simulink model "Dyn_6DoF_v2_0_R2015B"  (R2015b)
settings: Solver=ode4  SolverMode=SingleTasking  StartTime=0.0  StopTime=simInit.TSIM  FixedStep=simInit.dt  MaxStep=simInit.dt  RelTol=1e-3
InitFcn:
  | close all
undefined symbols (not defined in the file): act, base_windspeed, constr, DE2019, DiscIntNeverNeededParam, ENVMT, Lbooth, loiterStates, omega_rate_max, params, simInit, T, winchParameter
libraries: simulink x41, simulink_extras x4, dspsigops x1
(part 5 of 6)

== matlab function Dyn_6DoF_v2_0_R2015B/AirborneSystem/6DoFDynamics/Subsystem/Estimations ==
  data: Ft input; F_a_B input; F_p_B input; v_k_B input; v_w_W input; mu_k output; Va output; mu_a output; alpha output; beta output; chi_a_dot_real output; gamma_a_dot_real output; M_OB input; longlat input; EULER input; pathangles_a output; pathangles_k output; v_k_O output; pos_W output; pos_O output; ENVMT parameter; DE2019 parameter; v_k_W output; h_tau input
% Copyright 2021 Delft University of Technology
%
% Licensed under the Apache License, Version 2.0 (the "License");
% you may not use this file except in compliance with the License.
% You may obtain a copy of the License at
%
%      http://www.apache.org/licenses/LICENSE-2.0
%
% Unless required by applicable law or agreed to in writing, software
% distributed under the License is distributed on an "AS IS" BASIS,
% WITHOUT WARRANTIES OR CONDITIONS OF ANY KIND, either express or implied.
% See the License for the specific language governing permissions and
% limitations under the License.

function [mu_k,Va, mu_a, alpha, beta, chi_a_dot_real,gamma_a_dot_real, ...
    pathangles_a, pathangles_k, v_k_O, pos_W, pos_O, v_k_W] = ...
    fcn(Ft, F_a_B, F_p_B, v_k_B, v_w_W,M_OB,longlat,EULER,...
    ENVMT, DE2019, h_tau)
%fcn - 6DoF dynamics estimations
%
% Inputs:
%    Ft      - Tether force magnitude at the kite
%    F_a_B   - Aerodynamic forces acting on kite in body reference frames
%    F_p_B   - Propulsion and brake forces acting on kite in body reference
%              frames 
%    v_k_B   - Kinetic velocity in body reference frame
%    M_OB    - Rotation matrix from body to inertial reference frame
%    longlat - Longtitude, latitude
%    EULER   - Euler angles
%    ENVMT   - Environment characteristics
%    DE2019  - Aircraft parameters
%    h_tau   - Height in tau reference frame
%
% Outputs:
%    mu_k              - Kinetic roll angle
%    Va                - Airspeed (magnitude)
%    mu_a              - Aerodynamic roll angle
%    alpha             - Pitch angle
%    beta              - Sideslip(yaw) angle
%    chi_a_dot_real    - rate of change in aerodynamic course heading
%    gamma_a_dot_real  - rate of change in aerodynamic path angle
%    pathangles_a      - Aerodynamic course heading and path angle
%    pathangles_k      - Kinetic course heading and path angle
%    v_k_O             - Kinetic velocity in inertial reference frame
%    pos_W             - Kite position in wind reference frame
%    pos_O             - Kite position in inertial reference frame
%    v_k_W             - Kinetic velocity in wind reference frame
%
% Author: Sebastian Rapp, Ph.D., Revised by: Dylan Eijkelhof, M.Sc.
% Delft University of Technology
% email address: d.eijkelhof@tudelft.nl
% December 2019; Last revision: 19-March-2021

%-------------	BEGIN CODE	--------------
% Preallocate variables
mu_k             = 0;
Va               = 0;
mu_a             = 0;
alpha            = 0; 
beta             = 0;
chi_a_dot_real   = 0;
gamma_a_dot_real = 0;
pathangles_a     = zeros(2,1);
pathangles_k     = zeros(2,1); 
M_B2ABar         = zeros(3,3);

long = longlat(1);
lat  = longlat(2);

M_WO = [cos(ENVMT.windDirection_rad), sin(ENVMT.windDirection_rad), 0;
        sin(ENVMT.windDirection_rad), -cos(ENVMT.windDirection_rad), 0;
        0, 0, -1];
    
pos_W = [cos(long)*cos(lat);
         sin(long)*cos(lat);
         sin(lat)]*abs(h_tau);
    
pos_O = M_WO'*pos_W;   
v_k_O = M_OB*v_k_B;
v_k_W =  M_WO*v_k_O;

v_a_W = v_k_W - v_w_W;
Va = norm(v_a_W);

v_a_O = transformFromWtoO(ENVMT.windDirection_rad, v_a_W);
v_a_B = M_OB' * v_a_O;

chi_k        = atan2( v_k_O(2), v_k_O(1) );
gamma_k      = -asin( v_k_O(3)/norm(v_k_O) );
pathangles_k = [chi_k; gamma_k];

chi_a        = atan2( v_a_O(2), v_a_O(1) );
gamma_a      = -asin( v_a_O(3)/norm(v_a_O) );
pathangles_a = [chi_a; gamma_a];

% Estimation of aerodynamic angles 
alpha = atan2( v_a_B(3), v_a_B(1) );
beta  = asin( v_a_B(2)/norm(v_a_B) );
mu_a  = asin( max( min( (cos(EULER(2))*sin(EULER(1)))/(cos(gamma_a)*cos(beta)) ...
    + tan(gamma_a) * tan(beta), 1),-1) ); 

beta_k = atan2( v_k_B(2), norm(v_k_B) );
mu_k   = asin( max( min( (cos(EULER(2))*sin(EULER(1)))/(cos(gamma_k)*cos(beta_k)) ...
    + tan(gamma_k) * tan(beta_k), 1),-1) ); 

c_m = cos(mu_a);
s_m = sin(mu_a);

c_a = cos(alpha);
s_a = sin(alpha);

c_b = cos(beta);
s_b = sin(beta);

M_B2ABar(1,1) = c_a*c_b;
M_B2ABar(1,2) = s_b;
M_B2ABar(1,3) = s_a*c_b;
M_B2ABar(2,1) = -c_a*s_b*c_m+s_a*s_m;
M_B2ABar(2,2) = c_b*c_m;
M_B2ABar(2,3) = -s_a*s_b*c_m-s_m*c_a;
M_B2ABar(3,1) = -c_a*s_b*s_m-s_a*c_m;
M_B2ABar(3,2) = c_b*s_m;
M_B2ABar(3,3) = -s_a*s_b*s_m+c_a*c_m;

% Estimtion of chi_a_dot and gamma_a_dot
c_chia = cos(chi_a);
s_chia = sin(chi_a);

c_gama = cos(gamma_a);
s_gama = sin(gamma_a);

M_ABar2O = zeros(3,3);

M_ABar2O(1,1) = c_chia*c_gama;
M_ABar2O(2,1) = s_chia*c_gama;
M_ABar2O(3,1) = -s_gama;
M_ABar2O(1,2) = -s_chia;
M_ABar2O(2,2) = c_chia;
M_ABar2O(3,2) = 0;
M_ABar2O(1,3) = c_chia*s_gama;
M_ABar2O(2,3) = s_chia*s_gama;
M_ABar2O(3,3) = c_gama;


F_g_t_Abar  = M_ABar2O' * ( [0;0;DE2019.mass*ENVMT.g] -Ft*pos_O/norm(pos_O) );
F_ap_B      = M_B2ABar * (F_a_B+F_p_B);
f_y         = F_ap_B(2) + F_g_t_Abar(2); 
f_z         = F_ap_B(3) + F_g_t_Abar(3);

chi_a_dot_real   = 1/cos(gamma_a)/Va/DE2019.mass  * (f_y);
gamma_a_dot_real = -1/Va/DE2019.mass * (f_z);

%-------------	END CODE	--------------
end

== matlab function Dyn_6DoF_v2_0_R2015B/AirborneSystem/6DoFDynamics/Subsystem/MATLAB Function2 ==
  data: v_k_B input; DE2019 parameter; F_a_B input; F_p_B input; ENVMT parameter; F_t_W input; Torques_B input; vel_k_W input; omega_OB_B input; longlat input; EULER input; h_tau input; vel_K_B_dot output; M_OB output; omega_OB_B_dot output; longlat_dot output; eta_EULER_dot output; h_tau_dot output
% Copyright 2021 Delft University of Technology
%
% Licensed under the Apache License, Version 2.0 (the "License");
% you may not use this file except in compliance with the License.
% You may obtain a copy of the License at
%
%      http://www.apache.org/licenses/LICENSE-2.0
%
% Unless required by applicable law or agreed to in writing, software
% distributed under the License is distributed on an "AS IS" BASIS,
% WITHOUT WARRANTIES OR CONDITIONS OF ANY KIND, either express or implied.
% See the License for the specific language governing permissions and
% limitations under the License.

function [vel_K_B_dot, M_OB, omega_OB_B_dot, longlat_dot, ...
    eta_EULER_dot, h_tau_dot] = fcn(v_k_B, DE2019, F_a_B, F_p_B ,...
    ENVMT, F_t_W, Torques_B, vel_k_W, omega_OB_B, longlat, EULER, h_tau)
%fcn - 6DoF dynamics
%
% Inputs:
%    v_k_B      - Kinetic velocity in body reference frame
%    DE2019     - Aircraft parameters
%    F_a_B      - Aerodynamic forces acting on kite in body reference frame
%    F_p_B      - Propulsion and brake forces acting on kite in body
%                 reference frame
%    ENVMT      - Environment characteristics
%    F_t_W      - Tether force pulling at the kite
%    Torques_B  - Roll, pitch and yaw moments in body reference frame
%    vel_k_W    - Kinetic velocity in wind reference frame
%    omega_OB_B - Roll, pitch and yaw rates
%    longlat    - Longtitude, latitude
%    EULER      - Euler angles
%    h_tau      - Height in tau reference frame
%
% Outputs:
%    vel_K_B_dot    - Rate of change in kinetic velocity in body reference
%                     frame
%    M_OB           - Rotation matrix from body to inertial reference frame
%    omega_OB_B_dot - Roll, pitch and yaw accellerations
%    longlat_dot    - Rate of change of longtitude, latitude
%    eta_EULER_dot	- Rate of change of euler angles
%    h_tau_dot      - Rate of change of height in tau reference frame
%
%
% Author: Sebastian Rapp, Ph.D., Revised by: Dylan Eijkelhof, M.Sc.
% Delft University of Technology
% email address: d.eijkelhof@tudelft.nl
% December 2019; Last revision: 19-March-2021

%-------------	BEGIN CODE	--------------
% Preallocate variables
omega_OB_B_dot = zeros(3,1);
eta_EULER_dot  = zeros(3,1);
longlat_dot    = zeros(2,1);
vel_K_B_dot    = zeros(3,1);

c_psi = cos(EULER(3));
s_psi = sin(EULER(3));

c_theta = cos(EULER(2));
s_theta = sin(EULER(2));

c_phi = cos(EULER(1));
s_phi = sin(EULER(1)); 

M_OB = [ c_psi*c_theta, c_psi*s_theta*s_phi-s_psi*c_phi, c_psi*s_theta*c_phi+s_psi*s_phi;
         s_psi*c_theta, s_psi*s_theta*s_phi+c_psi*c_phi, s_psi*s_theta*c_phi-c_psi*s_phi;
        -s_theta, c_theta*s_phi, c_theta*c_phi];

long = longlat(1);
lat  = longlat(2);

F_g_O = [0;0;DE2019.mass*ENVMT.g];
F_t_O = transformFromOtoW( ENVMT.windDirection_rad, F_t_W);

%Forces to body fixed frame
F_g_t_B  = M_OB'*(F_g_O+F_t_O); 
Forces_B = F_a_B + F_g_t_B + F_p_B ;

p=omega_OB_B(1);
q=omega_OB_B(2);
r=omega_OB_B(3);

u=v_k_B(1);
v=v_k_B(2);
w=v_k_B(3);
vel_K_B_dot = [r*v-q*w + 1/DE2019.mass * Forces_B(1);
               p*w-r*u + 1/DE2019.mass * Forces_B(2);
               q*u-p*v + 1/DE2019.mass * Forces_B(3)];

c_theta = cos(EULER(2));
s_theta = sin(EULER(2));

c_phi = cos(EULER(1));
s_phi = sin(EULER(1)); 

eta_EULER_dot = [1 s_phi*s_theta/c_theta c_phi*s_theta/c_theta;
                 0 c_phi -s_phi; 
                 0 s_phi/c_theta c_phi/c_theta]*omega_OB_B;

Gamma  = DE2019.Jx*DE2019.Jz-DE2019.Jxz^2;
Gamma1 = (DE2019.Jxz*(DE2019.Jx - DE2019.Jy + DE2019.Jz ))/Gamma;
Gamma2 = (DE2019.Jz * (DE2019.Jz - DE2019.Jy) + DE2019.Jxz^2)/Gamma;
Gamma3 = DE2019.Jz/Gamma;
Gamma4 = DE2019.Jxz/Gamma;
Gamma5 = (DE2019.Jz - DE2019.Jx)/DE2019.Jy;
Gamma6 = DE2019.Jxz / DE2019.Jy;
Gamma7 = ((DE2019.Jx - DE2019.Jy)*DE2019.Jx + DE2019.Jxz^2 )/Gamma;
Gamma8 = DE2019.Jx / Gamma;

omega_OB_B_dot = [Gamma1 * p * q - Gamma2 * q * r + Gamma3 * Torques_B(1) + Gamma4 * Torques_B(3);
    Gamma5 * p * r - Gamma6 * (p^2 - r^2) + 1/DE2019.Jy *Torques_B(2);
     Gamma7 * p * q - Gamma1 * q * r + Gamma4 * Torques_B(1) + Gamma8 * Torques_B(3)];

%% Position propagation
sin_lat  = sin(lat);
sin_long = sin(long);
cos_lat  = cos(lat);
cos_long = cos(long);
 
M_tauW = [-sin_lat*cos_long, -sin_lat*sin_long,cos_lat;
    -sin_long, cos_long, 0;
    -cos_lat*cos_long, -cos_lat*sin_long, -sin_lat];

v_k_tau = M_tauW*vel_k_W;

long_dot = v_k_tau(2)/( abs(h_tau)*cos(lat));
lat_dot  = v_k_tau(1)/abs(h_tau);

h_tau_dot = -v_k_tau(3);

longlat_dot = [long_dot;
               lat_dot];

%-------------	END CODE	--------------
end

== matlab function Dyn_6DoF_v2_0_R2015B/AirborneSystem/FlightControlSystem/AttitudeAndRateLoop/AttitudeController/InversionAttitude ==
  data: omega_OB_B_cmd output size=[3,1]; mu_a input size=1; alpha input size=1; beta input size=1; nu_mu_a input size=1; nu_alpha_a input size=1; nu_beta_a input size=1; chi_a_dot_real input size=1; gamma_a_dot_real input size=1; gamma_a input; nu_hat output; constr parameter
% Copyright 2021 Delft University of Technology
%
% Licensed under the Apache License, Version 2.0 (the "License");
% you may not use this file except in compliance with the License.
% You may obtain a copy of the License at
%
%      http://www.apache.org/licenses/LICENSE-2.0
%
% Unless required by applicable law or agreed to in writing, software
% distributed under the License is distributed on an "AS IS" BASIS,
% WITHOUT WARRANTIES OR CONDITIONS OF ANY KIND, either express or implied.
% See the License for the specific language governing permissions and
% limitations under the License.

function [omega_OB_B_cmd, nu_hat]  = Attitude_inv( mu_a, alpha, beta, nu_mu_a,...
                                    nu_alpha_a, nu_beta_a, chi_a_dot_real,...
                                    gamma_a_dot_real, gamma_a, constr)
%Attitude_inv - Inverse attitude from error to actual
%
% Inputs:
%    mu_a               - Actual roll angle
%    alpha              - Actual pitch angle
%    beta               - Actual yaw angle
%    nu_mu_a            - Roll angle error w.r.t. actual with controller gains
%    nu_alpha_a         - Pitch angle error w.r.t. actual with controller gains
%    nu_beta_a          - Yaw angle error w.r.t. actual with controller gains
%    chi_a_dot_real     - Rate of change of course heading
%    gamma_a_dot_real   - Rate of change of path angle
%    gamma_a            - Actual aerodynamic path angle
%    constr             - Aircraft manoeuvre constraints
%
% Outputs:
%    omega_OB_B_cmd     - Commanded roll, pitch and yaw rates
%    nu_hat             - Expected error
%
%
% Author: Sebastian Rapp, Ph.D., Revised by: Dylan Eijkelhof, M.Sc.
% Delft University of Technology
% email address: d.eijkelhof@tudelft.nl
% December 2019; Last revision: 19-March-2021

%-------------	BEGIN CODE	--------------

c_m = cos(mu_a);
s_m = sin(mu_a);

c_a = cos(alpha);
s_a = sin(alpha);

c_b = cos(beta);
s_b = sin(beta);

M_B2ABar = zeros(3,3);

M_B2ABar(1,1) = c_a*c_b;
M_B2ABar(1,2) = s_b;
M_B2ABar(1,3) = s_a*c_b;
M_B2ABar(2,1) = -c_a*s_b*c_m+s_a*s_m;
M_B2ABar(2,2) = c_b*c_m;
M_B2ABar(2,3) = -s_a*s_b*c_m-s_m*c_a;
M_B2ABar(3,1) = -c_a*s_b*s_m-s_a*c_m;
M_B2ABar(3,2) = c_b*s_m;
M_B2ABar(3,3) = -s_a*s_b*s_m+c_a*c_m;


%% Inversion 

omega_OAbar_Abar = [-chi_a_dot_real*sin(gamma_a); 
                     gamma_a_dot_real; 
                     chi_a_dot_real*cos(gamma_a)];
                 
omega_OAbar_B = M_B2ABar'*omega_OAbar_Abar;
omega_OB_B_cmd =  [cos(alpha)*cos(beta) * nu_mu_a + nu_beta_a*sin(alpha); 
                  sin(beta)*nu_mu_a+nu_alpha_a;
                    sin(alpha)*cos(beta)*nu_mu_a - cos(alpha)*nu_beta_a] + omega_OAbar_B;

omega_OB_B_cmd_sat = max( min( omega_OB_B_cmd , constr.max_rates_B), -constr.max_rates_B ); 

% Expected pseudo-control
omega_AB_B = omega_OB_B_cmd_sat - M_B2ABar'*( [-chi_a_dot_real*sin(gamma_a);
                         gamma_a_dot_real; 
                         chi_a_dot_real*cos(gamma_a)]);
nu_x_hat = ( c_a*omega_AB_B(1) + s_a * omega_AB_B(3)  )/cos( beta );
nu_y_hat = -s_b*nu_x_hat  + omega_AB_B(2); 
nu_z_hat = ( omega_AB_B(1)*s_a - omega_AB_B(3) * c_a );
nu_hat = [nu_x_hat; nu_y_hat; nu_z_hat];

end

== matlab function Dyn_6DoF_v2_0_R2015B/AirborneSystem/FlightControlSystem/AttitudeAndRateLoop/RateLoop/ControlAllocation/allocation ==
  data: dC_pqr input; Delta_deltas output; alpha input; DE2019 parameter
% Copyright 2021 Delft University of Technology
%
% Licensed under the Apache License, Version 2.0 (the "License");
% you may not use this file except in compliance with the License.
% You may obtain a copy of the License at
%
%      http://www.apache.org/licenses/LICENSE-2.0
%
% Unless required by applicable law or agreed to in writing, software
% distributed under the License is distributed on an "AS IS" BASIS,
% WITHOUT WARRANTIES OR CONDITIONS OF ANY KIND, either express or implied.
% See the License for the specific language governing permissions and
% limitations under the License.

function Delta_deltas = fcn(dC_pqr, alpha, DE2019)
%Attitude_inv - Allocation matrix from moment increments to surface increments.
%
% Inputs:
%    dC_pqr        - Delta roll, pitch and yaw coefficients
%    alpha         - Actual pitch angle
%    DE2019        - Aircraft parameters
%
% Outputs:
%    Delta_deltas  - Delta actuator deflections
%
% Author: Sebastian Rapp, Ph.D., Revised by: Dylan Eijkelhof, M.Sc.
% Delft University of Technology
% email address: d.eijkelhof@tudelft.nl
% December 2019; Last revision: 19-March-2021

%-------------	BEGIN CODE	--------------
 
Cl_deltaA =DE2019.Cl_deltaA_0 + DE2019.Cl_deltaA_alpha * alpha + DE2019.Cl_deltaA_alpha2 * alpha^2;
Cl_deltaR =DE2019.Cl_deltaR_0 + DE2019.Cl_deltaR_alpha * alpha + DE2019.Cl_deltaR_alpha2 * alpha^2;                                 
 
Cm_deltaA =DE2019.Cm_deltaA_0 + DE2019.Cm_deltaA_alpha * alpha + DE2019.Cm_deltaA_alpha2 * alpha^2;  
Cm_deltaE = DE2019.Cm_deltaE_0  + DE2019.Cm_deltaE_alpha * alpha + DE2019.Cm_deltaE_alpha2 * alpha^2; 
 
Cn_deltaA =DE2019.Cn_deltaA_0 + DE2019.Cn_deltaA_alpha * alpha + DE2019.Cn_deltaA_alpha2 * alpha^2;  
Cn_deltaR =DE2019.Cn_deltaR_0 + DE2019.Cn_deltaR_alpha * alpha + DE2019.Cn_deltaR_alpha2 * alpha^2;
 
Ba = [[Cl_deltaA,0,Cl_deltaR];[Cm_deltaA,Cm_deltaE,0];[Cn_deltaA,0,Cn_deltaR]];
 
Delta_deltas = Ba\dC_pqr;

%-------------	END CODE	--------------
 
end

== matlab function Dyn_6DoF_v2_0_R2015B/AirborneSystem/ForcesAndTorques/aerodynamic forces FSI/Wing Aero/If Action Subsystem/MATLAB Function ==
  data: u input; y output
% Copyright 2021 Delft University of Technology
%
% Licensed under the Apache License, Version 2.0 (the "License");
% you may not use this file except in compliance with the License.
% You may obtain a copy of the License at
%
%      http://www.apache.org/licenses/LICENSE-2.0
%
% Unless required by applicable law or agreed to in writing, software
% distributed under the License is distributed on an "AS IS" BASIS,
% WITHOUT WARRANTIES OR CONDITIONS OF ANY KIND, either express or implied.
% See the License for the specific language governing permissions and
% limitations under the License.

function y = placeholder(u)

y = zeros(6,1);

== matlab function Dyn_6DoF_v2_0_R2015B/RequirementModelsAndLogging/MATLAB Function ==
  data: time input; eul input; stop_flag output; eul_old input
% Copyright 2021 Delft University of Technology
%
% Licensed under the Apache License, Version 2.0 (the "License");
% you may not use this file except in compliance with the License.
% You may obtain a copy of the License at
%
%      http://www.apache.org/licenses/LICENSE-2.0
%
% Unless required by applicable law or agreed to in writing, software
% distributed under the License is distributed on an "AS IS" BASIS,
% WITHOUT WARRANTIES OR CONDITIONS OF ANY KIND, either express or implied.
% See the License for the specific language governing permissions and
% limitations under the License.

function stop_flag = fcn(time, eul,eul_old)
phi = eul(1);
theta = eul(2);
% psi = eul(3);

phi_old = eul_old(1);
theta_old = eul_old(2);
% psi_old = eul_old(3);

if time>40
    if ((phi>pi/2 || phi<-pi/2) && sign(phi) ~= sign(phi_old))
        stop_flag = 1;
    elseif ((theta>pi/2 || theta<-pi/2) && sign(theta) ~= sign(theta_old))
        stop_flag = 1; 
%     elseif ((psi>pi/2 || psi<-pi/2) && sign(psi) ~= sign(psi_old))
%         stop_flag = 1; 
    else
        stop_flag = 0;
    end
else
    stop_flag = 0;
end
end

== matlab function Dyn_6DoF_v2_0_R2015B/RequirementModelsAndLogging/MATLAB Function1 ==
  data: Lift output; F_a_B input; Drag output; AoA input
% Copyright 2021 Delft University of Technology
%
% Licensed under the Apache License, Version 2.0 (the "License");
% you may not use this file except in compliance with the License.
% You may obtain a copy of the License at
%
%      http://www.apache.org/licenses/LICENSE-2.0
%
% Unless required by applicable law or agreed to in writing, software
% distributed under the License is distributed on an "AS IS" BASIS,
% WITHOUT WARRANTIES OR CONDITIONS OF ANY KIND, either express or implied.
% See the License for the specific language governing permissions and
% limitations under the License.

function [Lift, Drag]  = estimate_drag(F_a_B, AoA)
%estimate_drag - Transform drag from B to A reference frame
%
% Inputs:
%    F_a_B     - Aerodynamic forces in body reference frame
%    AoA       - Angle of Attack
%
% Outputs:
%    Drag    - Drag force
%
% Example: 
%    [Drag] = estimate_drag(F_a_B, AoA)
%
% Author: Sebastian Rapp, Ph.D., Revised by: Dylan Eijkelhof, M.Sc.
% Delft University of Technology
% email address: s.rapp@tudelft.nl
% email address: d.eijkelhof@tudelft.nl
% December 2019; Last revision: 06-October-2020

%-------------	BEGIN CODE	--------------

F_a_A = [cos(AoA), 0, sin(AoA);
    0, 1, 0; 
    -sin(AoA), 0, cos(AoA)] * F_a_B;

Lift = -F_a_A(3);
Drag = -F_a_A(1);

%-------------	 END CODE	--------------

end

== matlab function Dyn_6DoF_v2_0_R2015B/AirborneSystem/FlightControlSystem/PathFollowingController_SS_3/FlightOnFlatEarth (Retraction&Loitering)/CalculateAttitudeCmds/FlightPathLoopRetraction_Aerodynamic/FlightpathReferenceModels/SecondOrderReferenceModel_course/wrapto2pi ==
  data: u input; y output
% Copyright 2021 Delft University of Technology
%
% Licensed under the Apache License, Version 2.0 (the "License");
% you may not use this file except in compliance with the License.
% You may obtain a copy of the License at
%
%      http://www.apache.org/licenses/LICENSE-2.0
%
% Unless required by applicable law or agreed to in writing, software
% distributed under the License is distributed on an "AS IS" BASIS,
% WITHOUT WARRANTIES OR CONDITIONS OF ANY KIND, either express or implied.
% See the License for the specific language governing permissions and
% limitations under the License.

function y = wrap_to_2pi(u)
u = mod(u, 2*pi); 
if u > pi 
    du = mod(u,pi);
    y = -pi+du; 
elseif u < -pi 
    du = mod(u,-pi); 
    y = pi+du;
else
    y = u; 
end
end

== matlab function Dyn_6DoF_v2_0_R2015B/Environment_SS_5/MATLAB Function1 ==
  data: v_w_u input; v_w_p_mat output
% Copyright 2021 Delft University of Technology
%
% Licensed under the Apache License, Version 2.0 (the "License");
% you may not use this file except in compliance with the License.
% You may obtain a copy of the License at
%
%      http://www.apache.org/licenses/LICENSE-2.0
%
% Unless required by applicable law or agreed to in writing, software
% distributed under the License is distributed on an "AS IS" BASIS,
% WITHOUT WARRANTIES OR CONDITIONS OF ANY KIND, either express or implied.
% See the License for the specific language governing permissions and
% limitations under the License.

function v_w_p_mat = fcn(v_w_u)

v_w_p_mat = zeros( 3, length( v_w_u) );
v_w_p_mat(1,:) = v_w_u';

== matlab function Dyn_6DoF_v2_0_R2015B/AirborneSystem/FlightControlSystem/AirspeedController_SS_1/Airspeed_Brake/FeedforwardPart ==
  data: gamma input; BF output; nu_V input; ENVMT parameter; Drag_force input; DE2019 parameter
% Copyright 2021 Delft University of Technology
%
% Licensed under the Apache License, Version 2.0 (the "License");
% you may not use this file except in compliance with the License.
% You may obtain a copy of the License at
%
%      http://www.apache.org/licenses/LICENSE-2.0
%
% Unless required by applicable law or agreed to in writing, software
% distributed under the License is distributed on an "AS IS" BASIS,
% WITHOUT WARRANTIES OR CONDITIONS OF ANY KIND, either express or implied.
% See the License for the specific language governing permissions and
% limitations under the License.

function BF = feedforward_brake(gamma, nu_V,  ENVMT, Drag_force, DE2019)
%feedforward_brake - Brake force calculation for velocity decrease
%
% Inputs:
%    gamma      - Path angle (glideslope)
%    nu_V       - Controlled velocity parameter
%    ENVMT      - Environmental characteristics
%    Drag_force	- Drag
%    DE2019     - Aircraft characteristics
%
% Outputs:
%    BF          - Brake force
%
% Example: 
%    BF = feedforward_thrust(gamma, nu_V,  ENVMT, Drag_force, DE2019)
%
% Author: Sebastian Rapp, Ph.D., Revised by: Dylan Eijkelhof, M.Sc.
% Delft University of Technology
% email address: s.rapp@tudelft.nl
% email address: d.eijkelhof@tudelft.nl
% December 2019; Last revision: 06-October-2020

%-------------	BEGIN CODE	--------------

BF = DE2019.mass * ( ENVMT.g * sin(gamma) + nu_V ) + Drag_force; % required thrust

%-------------	 END CODE	--------------
end

== stateflow chart Dyn_6DoF_v2_0_R2015B/GroundSystem_SS_6/GroundControl/Select_init_sol_for_pathfollowing ==
  state Init
    entry: sol_init = x;
  state Pumping
    entry: sol_init = transition_phi;
  (default) -> Init
  Init -> Pumping : [fm == 6]
  data: x input; fm input; sol_init output; transition_phi input

== matlab function Dyn_6DoF_v2_0_R2015B/AirborneSystem/FlightControlSystem/AirspeedController_SS_1/Airspeed_Brake/MATLAB Function ==
  data: F_a_B input; Drag output; AoA input
% Copyright 2021 Delft University of Technology
%
% Licensed under the Apache License, Version 2.0 (the "License");
% you may not use this file except in compliance with the License.
% You may obtain a copy of the License at
%
%      http://www.apache.org/licenses/LICENSE-2.0
%
% Unless required by applicable law or agreed to in writing, software
% distributed under the License is distributed on an "AS IS" BASIS,
% WITHOUT WARRANTIES OR CONDITIONS OF ANY KIND, either express or implied.
% See the License for the specific language governing permissions and
% limitations under the License.

function Drag  = estimate_drag(F_a_B, AoA)
%estimate_drag - Transform drag from B to A reference frame
%
% Inputs:
%    F_a_B     - Aerodynamic forces in body reference frame
%    AoA       - Angle of Attack
%
% Outputs:
%    Drag    - Drag force
%
% Example: 
%    [Drag] = estimate_drag(F_a_B, AoA)
%
% Author: Sebastian Rapp, Ph.D., Revised by: Dylan Eijkelhof, M.Sc.
% Delft University of Technology
% email address: s.rapp@tudelft.nl
% email address: d.eijkelhof@tudelft.nl
% December 2019; Last revision: 06-October-2020

%-------------	BEGIN CODE	--------------

F_a_A = [cos(AoA), 0, sin(AoA);
    0, 1, 0; 
    -sin(AoA), 0, cos(AoA)] * F_a_B;

Drag = -F_a_A(1);

%-------------	 END CODE	--------------

end

== matlab function Dyn_6DoF_v2_0_R2015B/AirborneSystem/FlightControlSystem/AirspeedController_SS_1/Airspeed_Brake/hedging ==
  data: Drag_force input; gamma input; nu_V output; BF input; ENVMT parameter; DE2019 parameter
% Copyright 2021 Delft University of Technology
%
% Licensed under the Apache License, Version 2.0 (the "License");
% you may not use this file except in compliance with the License.
% You may obtain a copy of the License at
%
%      http://www.apache.org/licenses/LICENSE-2.0
%
% Unless required by applicable law or agreed to in writing, software
% distributed under the License is distributed on an "AS IS" BASIS,
% WITHOUT WARRANTIES OR CONDITIONS OF ANY KIND, either express or implied.
% See the License for the specific language governing permissions and
% limitations under the License.

function nu_V = hedgingV(Drag_force, gamma, BF, ENVMT, DE2019)

%hedgingV
%
% Inputs:
%    Drag_force	- Drag
%    gamma      - Path angle (glideslope)
%    BF         - Brake force
%    ENVMT      - Environmental characteristics
%    DE2019     - Aircraft characteristics
%
% Outputs:
%    nu_V       - Controlled velocity parameter
%
% Example: 
%    nu_V = hedgingV(Drag_force, gamma, BF, ENVMT, DE2019)
%
% Author: Sebastian Rapp, Ph.D., Revised by: Dylan Eijkelhof, M.Sc.
% Delft University of Technology
% email address: s.rapp@tudelft.nl
% email address: d.eijkelhof@tudelft.nl
% December 2019; Last revision: 06-October-2020

%-------------	BEGIN CODE	--------------

nu_V = (BF-Drag_force)/DE2019.mass - ENVMT.g * sin(gamma); 

%-------------	 END CODE	--------------
end

== matlab function Dyn_6DoF_v2_0_R2015B/AirborneSystem/FlightControlSystem/AirspeedController_SS_1/Airspeed_Control/FeedforwardPart ==
  data: gamma input; T output; nu_V input; ENVMT parameter; Drag_force input; DE2019 parameter
% Copyright 2021 Delft University of Technology
%
% Licensed under the Apache License, Version 2.0 (the "License");
% you may not use this file except in compliance with the License.
% You may obtain a copy of the License at
%
%      http://www.apache.org/licenses/LICENSE-2.0
%
% Unless required by applicable law or agreed to in writing, software
% distributed under the License is distributed on an "AS IS" BASIS,
% WITHOUT WARRANTIES OR CONDITIONS OF ANY KIND, either express or implied.
% See the License for the specific language governing permissions and
% limitations under the License.

function T = feedforward_thrust(gamma, nu_V,  ENVMT, Drag_force, DE2019)
%feedforward_thrust - Thrust calculation for velocity initialisation
%
% Inputs:
%    gamma      - Path angle (glideslope)
%    nu_V       - Controlled velocity parameter
%    ENVMT      - Environmental characteristics
%    Drag_force	- Drag
%    DE2019     - Aircraft characteristics
%
% Outputs:
%    T          - Thrust force
%
% Example: 
%    T = feedforward_thrust(gamma, nu_V,  ENVMT, Drag_force, DE2019)
%
% Author: Sebastian Rapp, Ph.D., Revised by: Dylan Eijkelhof, M.Sc.
% Delft University of Technology
% email address: s.rapp@tudelft.nl
% email address: d.eijkelhof@tudelft.nl
% December 2019; Last revision: 06-October-2020

%-------------	BEGIN CODE	--------------

T = DE2019.mass * ( ENVMT.g * sin(gamma) + nu_V ) + Drag_force; % required thrust

% Based on the quotient of commmanded to max. available thrust
% F_T_max = ENVMT.rhos * DE2019.S_prop * DE2019.C_prop * DE2019.k_motor * (DE2019.k_motor - Va);
% delta_t = T/F_T_max; 

%-------------	 END CODE	--------------
end

== matlab function Dyn_6DoF_v2_0_R2015B/AirborneSystem/FlightControlSystem/AirspeedController_SS_1/Airspeed_Control/MATLAB Function ==
  data: F_a_B input; Drag output; AoA input
% Copyright 2021 Delft University of Technology
%
% Licensed under the Apache License, Version 2.0 (the "License");
% you may not use this file except in compliance with the License.
% You may obtain a copy of the License at
%
%      http://www.apache.org/licenses/LICENSE-2.0
%
% Unless required by applicable law or agreed to in writing, software
% distributed under the License is distributed on an "AS IS" BASIS,
% WITHOUT WARRANTIES OR CONDITIONS OF ANY KIND, either express or implied.
% See the License for the specific language governing permissions and
% limitations under the License.

function Drag = estimate_drag(F_a_B, AoA)

%estimate_drag - Transform drag from B to A reference frame
%
% Inputs:
%    F_a_B     - Aerodynamic forces in body reference frame
%    AoA       - Angle of Attack
%
% Outputs:
%    Drag    - Drag force
%
% Example: 
%    Drag = estimate_drag(F_a_B, AoA)
%
% Author: Sebastian Rapp, Ph.D., Revised by: Dylan Eijkelhof, M.Sc.
% Delft University of Technology
% email address: s.rapp@tudelft.nl
% email address: d.eijkelhof@tudelft.nl
% December 2019; Last revision: 06-October-2020

%-------------	BEGIN CODE	--------------

F_a_A = [cos(AoA), 0, sin(AoA);
    0, 1, 0; 
    -sin(AoA), 0, cos(AoA)] * F_a_B;

Drag = -F_a_A(1);

%-------------	 END CODE	--------------
end

== matlab function Dyn_6DoF_v2_0_R2015B/AirborneSystem/FlightControlSystem/AirspeedController_SS_1/Airspeed_Control/hedging ==
  data: Drag_force input; gamma input; nu_V output; T input; ENVMT parameter; DE2019 parameter
% Copyright 2021 Delft University of Technology
%
% Licensed under the Apache License, Version 2.0 (the "License");
% you may not use this file except in compliance with the License.
% You may obtain a copy of the License at
%
%      http://www.apache.org/licenses/LICENSE-2.0
%
% Unless required by applicable law or agreed to in writing, software
% distributed under the License is distributed on an "AS IS" BASIS,
% WITHOUT WARRANTIES OR CONDITIONS OF ANY KIND, either express or implied.
% See the License for the specific language governing permissions and
% limitations under the License.

function nu_V = hedgingV(Drag_force, gamma, T, ENVMT, DE2019)

%hedgingV
%
% Inputs:
%    Drag_force	- Drag
%    gamma      - Path angle (glideslope)
%    T          - Thrust force
%    ENVMT      - Environmental characteristics
%    DE2019     - Aircraft characteristics
%
% Outputs:
%    nu_V       - Controlled velocity parameter
%
% Example: 
%    nu_V = hedgingV(Drag_force, gamma, T, ENVMT, DE2019)
%
% Author: Sebastian Rapp, Ph.D., Revised by: Dylan Eijkelhof, M.Sc.
% Delft University of Technology
% email address: s.rapp@tudelft.nl
% email address: d.eijkelhof@tudelft.nl
% December 2019; Last revision: 06-October-2020

%-------------	BEGIN CODE	--------------

% Based on the quotient of commmanded to max. available thrust
% F_T_max = ENVMT.rhos * DE2019.S_prop * DE2019.C_prop * DE2019.k_motor * (DE2019.k_motor - Va);
% T = F_T_max * delta_t; 

nu_V = (T-Drag_force)/DE2019.mass - ENVMT.g * sin(gamma); 

%-------------	 END CODE	--------------
end

== stateflow chart Dyn_6DoF_v2_0_R2015B/GroundSystem_SS_6/StateMachine/StateMachine ==
  state loiter
    entry: flightMode = 1;
    during: F_t_set = Ft_set_loiter;
    entry: init_throttle_flag = 1;
    entry: sub_flight_state = 1;
  state Traction4 % slowly increase tether force
    entry: flightMode=5;
    during: F_t_set = calcSetpoint(alpha2,Ft_set_prev,Ft_set_loiter);
    exit: init_throttle_flag = 1;
    entry: sub_flight_state = 2;
  note: F_t_m>F_set_retraction
  note: pos_x_W<x_trigger_transition
  state Retraction3 [commented out]
    entry: flightMode=6;
    entry: F_t_set =calcSetpoint(1,Ft_set_prev,3000);
    %entry: F_t_set = 0;
    entry: reelin_flag = 1;
    entry: sub_flight_state = 8;
    entry: path_captured_flag = 0;
  state Traction2 % slowly increase tether force
    entry: flightMode=5;
    during: F_t_set = calcSetpoint(alpha2,Ft_set_prev,F_T_traction_set);
    exit: init_throttle_flag = 1;
    entry: sub_flight_state = 2;
  state Retraction1
    entry: flightMode=6;
    entry: F_t_set =calcSetpoint(alpha2,F_set_retraction,Ft_set_prev);
    entry: reelin_flag = 1;
    entry: sub_flight_state = 7;
    entry: path_captured_flag = 0;
  state Retraction
    entry: flightMode=6;
    entry: reelin_flag = 1;
    during: F_t_set = calcSetpoint(alpha2,F_set_retraction,Ft_set_prev);
    entry: sub_flight_state = 6;
  state Traction1
    entry: flightMode=5;
    during: F_t_set = calcSetpoint(alpha2,Ft_set_prev,F_T_traction_set);
    entry: sub_flight_state = 3;
  state Traction3
    entry: flightMode=5;
    entry: path_captured_flag = 1;
    entry: init_throttle_flag = 0;
    during: F_t_set = calcSetpoint(alpha2,Ft_set_prev,F_T_traction_set);
    entry: sub_flight_state = 4;
  state Trans2Retract
    entry: flightMode=5;
    during: F_t_set = calcSetpoint(alpha2,Ft_set_prev,F_T_traction_set);
    entry: sub_flight_state = 5;
  (default) -> loiter
  loiter -> Traction4 % slowly increase tether force : [trigger_kite_mode == 1]
  Traction4 % slowly increase tether force -> Traction2 % slowly increase tether force : [pre_pc_mode_flag==0]
  Retraction1 -> Retraction3 [commented out] : [x_trigger_transition>0]
  Retraction1 -> Traction1 : [pos_x_W<x_trigger_transition]
  Traction2 % slowly increase tether force -> Traction3 : [long_kite>0]
  Retraction -> Retraction1 : [F_t_m<1.1*F_set_retraction]
  (junction 286) -> Retraction
  Traction1 -> Traction3 : [cross_track_error < crosstrackerror_condition&&Va>=Vamin]
  Traction3 -> Trans2Retract : [(l_t>l_t_max||init_retraction_flag)]
  Traction3 -> Trans2Retract [commented out] : [(l_t>l_t_max||init_retraction_flag)&& (path_parameter_s >= (5*pi/3+.5*pi/180) && path_parameter_s <=5*pi/3+1*pi/180)]
  Traction3 -> Trans2Retract [commented out] : [(l_t>l_t_max||init_retraction_flag)&& (path_parameter_s >= (2*pi/3+.5*pi/180) && path_parameter_s <= 2*pi/3+1*pi/180)]
  Trans2Retract -> (junction 286) [order 1] : [path_parameter_s >= (pi/2+.5*pi/180) && path_parameter_s <= pi/2+1*pi/180]
  (junction 319) -> (junction 286)
  Trans2Retract -> (junction 319) [order 2] : [path_parameter_s >= (3*pi/2+.5*pi/180) && path_parameter_s <=3*pi/2+1*pi/180]
  (junction 348) -> (junction 319) [commented out]
  Trans2Retract -> (junction 348) [commented out] : [Chi >= (0-0.5*pi/180) && Chi <= 0+0.5*pi/180]
  data: Ft_set function_output; alpha1_ function_input; Ft_set_prev_ function_input; F_T_traction_set_ function_input; flightMode output; long_kite input; lat_kite input; l_t input; F_t input; Lbooth parameter; pos_x_W input; pos_y_W input; F_t_set output; F_T_traction_set parameter double; F_set_retraction parameter; a_booth parameter; b_booth parameter; l_t_min parameter; lat_trans parameter; l_t_max parameter; Ft_set_prev input; alpha2 parameter; Va input; lat_init input; traction_trigger input; cross_track_error input; trigger_kite_mode input; init_throttle_flag output size=1; crosstrackerror_condition parameter; Vamin parameter; init_retraction_flag input; Ft_set_loiter parameter; phi0 input; F_t_m input; sub_flight_state output =1; pre_pc_mode_flag input; path_parameter_s input; sim_time input; reelin_flag local; path_captured_flag local; x_trigger_transition input; side local; Chi input
  function Ft_set = calcSetpoint(alpha1_,Ft_set_prev_, F_T_traction_set_):
    | % Copyright 2020 Delft University of Technology
    | %
    | % Licensed under the Apache License, Version 2.0 (the "License");
    | % you may not use this file except in compliance with the License.
    | % You may obtain a copy of the License at
    | %
    | %      http://www.apache.org/licenses/LICENSE-2.0
    | %
    | % Unless required by applicable law or agreed to in writing, software
    | % distributed under the License is distributed on an "AS IS" BASIS,
    | % WITHOUT WARRANTIES OR CONDITIONS OF ANY KIND, either express or implied.
    | % See the License for the specific language governing permissions and
    | % limitations under the License. 
    | 
    | function Ft_set = calcSetpoint(alpha1_,Ft_set_prev_, F_T_traction_set_)
    |  
    | Ft_set =  alpha1_ * F_T_traction_set_ +(1-alpha1_)*Ft_set_prev_;
    | 
    | end

== stateflow chart Dyn_6DoF_v2_0_R2015B/AirborneSystem/FlightControlSystem/AirspeedController_SS_1/Chart ==
  state Throttle_Off
    entry: throttle_on = 0;
  state Throttle_On
    entry: throttle_on = 1;
  (default) -> Throttle_Off
  Throttle_Off -> Throttle_On : [Va<Va_min || manual_switch_on || init_throttle_flag]
  Throttle_On -> Throttle_Off : [Va>Va_min+10&&manual_switch_on==0&& init_throttle_flag ==0]
  data: Va input; Va_min input; init_throttle_flag input; throttle_on output; manual_switch_on input

== matlab function Dyn_6DoF_v2_0_R2015B/Visualisation/Visualisation ==
  settings: updateMethod=DISCRETE  sampleTime=sample_time_vis
  data: t input; p_t_x input; p_t_y input; p_t_z input; phi0_update input; pos_O input; eta_OB input; params parameter; ENVMT parameter; sub_flight_state input; arcP input; sampletime input
% Copyright 2021 Delft University of Technology
%
% Licensed under the Apache License, Version 2.0 (the "License");
% you may not use this file except in compliance with the License.
% You may obtain a copy of the License at
%
%      http://www.apache.org/licenses/LICENSE-2.0
%
% Unless required by applicable law or agreed to in writing, software
% distributed under the License is distributed on an "AS IS" BASIS,
% WITHOUT WARRANTIES OR CONDITIONS OF ANY KIND, either express or implied.
% See the License for the specific language governing permissions and
% limitations under the License.

function Visualisation(t,p_t_x,p_t_y,p_t_z,phi0_update, pos_O,eta_OB,params, ENVMT, sub_flight_state, arcP, sampletime)   
    persistent handleTether
    persistent pathpoints
    persistent referencePath
    persistent Vert
    persistent handlePlane
    persistent retractionPath
    
    coder.extrinsic('plot3','patch','animatedline','addpoints');
 
    %% Figure settings
    if t==0
        figure(99)
%         addToolbarExplorationButtons(gcf)
        xlabel('x_W (m)');%, 'interpreter', 'latex')
        ylabel('y_W (m)');%, 'interpreter', 'latex')
        zlabel('z_W (m)');%, 'interpreter', 'latex')

        grid on
        box on;
        axis equal; hold on;

        view(30,21); % set the vieew angle for figure

        ax = [-500 1500];
        ay = [-1000 1000];
        az = [0 1200];
        axis([ax,ay,az]);  hold on

        X = [ax(1);ax(2);ax(2);ax(1)];
        Y = [ay(1);ay(1);ay(2);ay(2)];
        Z = [0;0;0;0];

        c = [0 1 0; % red
        0 1 0; % green
        0 1 0;
        0 1 0];
        fill3(X,Y,Z, c(:,2),'EdgeColor','none','FaceColor',c(1,:),'FaceAlpha',0.1);
    end
    
    %% Draw tether particles
    if isempty(handleTether)
 
        M_WO = [cos(ENVMT.windDirection_rad), sin(ENVMT.windDirection_rad), 0;
        sin(ENVMT.windDirection_rad), -cos(ENVMT.windDirection_rad), 0;
        0, 0, -1];
        pos_W = M_WO*[pos_O(1);pos_O(2);pos_O(3)];
        handleTether = plot3( [0;flipud(p_t_x);pos_W(1)], [0;flipud(p_t_y);pos_W(2)],[0;flipud(p_t_z);pos_W(3)],...
            '-', 'color', [0.1 0.1 0.1], 'Markersize',2, 'Linewidth', 1.2,...
            'MarkerFaceColor', [0.3 0.3 0.3]); hold on;
    end
    
    %% Draw aircraft
    if isempty(handlePlane)
        pn = pos_O(1);
        pe = pos_O(2);
        pd = pos_O(3);
        phi = eta_OB(1);
        theta = eta_OB(2);
        psi = eta_OB(3);
        
        M_WO = [cos(ENVMT.windDirection_rad), sin(ENVMT.windDirection_rad), 0;
        sin(ENVMT.windDirection_rad), -cos(ENVMT.windDirection_rad), 0;
        0, 0, -1];
        
        scale = 6;
%         [F, Vert, C] = rndread('plane_thesis_big.stl');
        Image_kite = coder.load('plane_image.mat','F','Verti','C');
        F = Image_kite.F;
        Verti = Image_kite.Verti;
        C = Image_kite.C;
        Vert = scale*Verti'; 
        V = [ cos(psi)*cos(theta) , cos(psi)*sin(phi)*sin(theta) - cos(phi)*sin(psi) , sin(phi)*sin(psi) + cos(phi)*cos(psi)*sin(theta);
            cos(theta)*sin(psi)   , cos(phi)*cos(psi) + sin(phi)*sin(psi)*sin(theta) , cos(phi)*sin(psi)*sin(theta) - cos(psi)*sin(phi);
               -sin(theta)        ,             cos(theta)*sin(phi)                  ,             cos(phi)*cos(theta)                 ]...
               * Vert;
        V = V + [pn*ones(1,size(V,2));pe*ones(1,size(V,2));pd*ones(1,size(V,2))];
        V = M_WO*V;
        col =  [ 57/255, 106/255, 177/255  ];
        handlePlane = patch('faces', F, 'vertices' ,V');
        set(handlePlane, 'facec', 'b');              % Set the face color (force it)
        set(handlePlane, 'FaceVertexCData', C);       % Set the color (from file)
        set(handlePlane, 'EdgeColor','none');
        set(handlePlane, 'FaceLighting', 'none');
        set(handlePlane, 'FaceColor', col );
    end
    
    %% Draw black thin trail behind kite
    if isempty(pathpoints)
        pathpoints = animatedline('Linestyle','-','color', [85/255, 85/255, 85/255 ], 'Linewidth', .5);
    end
    
    %% Draw red target figure of 8 (traction)
    if isempty(referencePath)
        
        Lbooth.a = params.a_booth*params.b_booth;
        Lbooth.b = params.b_booth;
        Lbooth.phi0 = phi0_update;
        
        s = 0 : 0.01 : 2*pi;
        l_tether = norm(pos_O);
        Lem.a = Lbooth.a/(l_tether); 
        Lem.b = Lbooth.b/(l_tether); 
        Lem.phi0 = Lbooth.phi0;
        long_P = Lem.b * sin(s) ./( 1+(Lem.a/Lem.b*cos(s)).^2 );
        lat_P =   Lem.a * sin(s).*cos(s) ./ ( 1+(Lem.a/Lem.b*cos(s)).^2 );
        p_P = [ cos(long_P).*cos(lat_P);sin(long_P).*cos(lat_P);sin(lat_P)]*l_tether;
        phi_p_mean = Lbooth.phi0;
        M_WP = [cos(phi_p_mean),0, -sin(phi_p_mean);0, 1, 0;  sin(phi_p_mean),0, cos(phi_p_mean)];
        p_W = M_WP * p_P;
        referencePath = plot3( p_W(1,:),p_W(2,:),p_W(3,:) , '-', 'color', [1 0.3 0.3],'Linewidth', 1.5);
    end
    
    %% Draw red retraction path (retraction)
    if isempty(retractionPath)
        retractionPath = plot3( arcP(1,:),arcP(2,:),arcP(3,:), '--', 'color', [1 0.3 0.3],'Linewidth', .5);
    end
    
    if (mod(t,sampletime)==0 && t~=0)
        %% Change each element on figure to current positions
        Lbooth.a = params.a_booth*params.b_booth;
        Lbooth.b = params.b_booth;
        Lbooth.phi0 = phi0_update;
        
        pn = pos_O(1);
        pe = pos_O(2);
        pd = pos_O(3);
        phi = eta_OB(1);
        theta = eta_OB(2);
        psi = eta_OB(3);
        
        M_WO = [cos(ENVMT.windDirection_rad), sin(ENVMT.windDirection_rad), 0;
        sin(ENVMT.windDirection_rad), -cos(ENVMT.windDirection_rad), 0;
        0, 0, -1];
        
        % Tether
        set(handleTether,'XData',[0;flipud(p_t_x);-pn], 'YData',[0;flipud(p_t_y);pe],'ZData',[0;flipud(p_t_z);-pd]);
        
        % Kite
        V = [ cos(psi)*cos(theta), cos(psi)*sin(phi)*sin(theta) - cos(phi)*sin(psi), sin(phi)*sin(psi) + cos(phi)*cos(psi)*sin(theta);
            cos(theta)*sin(psi), cos(phi)*cos(psi) + sin(phi)*sin(psi)*sin(theta), cos(phi)*sin(psi)*sin(theta) - cos(psi)*sin(phi);
            -sin(theta),                              cos(theta)*sin(phi),                              cos(phi)*cos(theta)] * Vert;
        V = V + [pn*ones(1,size(V,2));pe*ones(1,size(V,2));pd*ones(1,size(V,2))];
        V = M_WO*V;
        set(handlePlane, 'Vertices', V');
        
        % Trail
        pos_W = M_WO*[pn;pe;pd];
        addpoints(pathpoints,pos_W(1), pos_W(2),pos_W(3))
        
        % Target figure (traction)
        s = 0 : 0.01 : 2*pi;
        l_tether = norm(pos_O);
        Lem.a = Lbooth.a/(l_tether); 
        Lem.b = Lbooth.b/(l_tether); 
        Lem.phi0 = Lbooth.phi0;
        long_P = Lem.b * sin(s) ./( 1+(Lem.a/Lem.b*cos(s)).^2 );
        lat_P =   Lem.a * sin(s).*cos(s) ./ ( 1+(Lem.a/Lem.b*cos(s)).^2 );
        p_P = [ cos(long_P).*cos(lat_P);sin(long_P).*cos(lat_P);sin(lat_P)]*l_tether;
        phi_p_mean = Lbooth.phi0;
        M_WP = [cos(phi_p_mean),0, -sin(phi_p_mean);0, 1, 0;  sin(phi_p_mean),0, cos(phi_p_mean)];
        p_W = M_WP * p_P;
        set(referencePath,'XData',p_W(1,:),'YData',p_W(2,:),'ZData',p_W(3,:));
        
        % Target path (retraction)
        if sub_flight_state >= 6
            set(retractionPath,'XData',arcP(1,:),'YData',arcP(2,:),'ZData',arcP(3,:));
        else
            set(retractionPath,'XData',zeros(1,size(arcP,2)),'YData',zeros(1,size(arcP,2)),'ZData',zeros(1,size(arcP,2)));
        end
    end

== stateflow chart Dyn_6DoF_v2_0_R2015B/AirborneSystem/FlightControlSystem/AirspeedController_SS_1/Chart1 ==
  state Throttle_Off
    entry: brake_on = 0;
  state Throttle_On
    entry: brake_on = 1;
  (default) -> Throttle_Off
  Throttle_Off -> Throttle_On : [(manual_switch_on || brake_flag) && Ft <= Ft_retract+3000 && Vk>Vk_min]
  Throttle_On -> Throttle_Off : [(manual_switch_on==0&& brake_flag ==0) || Vk<Vk_min]
  data: brake_flag input; Vk input; brake_on output; manual_switch_on input; Ft input; Ft_retract parameter; Vk_min parameter

== matlab function Dyn_6DoF_v2_0_R2015B/AirborneSystem/FlightControlSystem/AirspeedController_SS_1/MATLAB Function1 ==
  data: vel_k_O input; vel_k_h_W output; ENVMT parameter
% Copyright 2021 Delft University of Technology
%
% Licensed under the Apache License, Version 2.0 (the "License");
% you may not use this file except in compliance with the License.
% You may obtain a copy of the License at
%
%      http://www.apache.org/licenses/LICENSE-2.0
%
% Unless required by applicable law or agreed to in writing, software
% distributed under the License is distributed on an "AS IS" BASIS,
% WITHOUT WARRANTIES OR CONDITIONS OF ANY KIND, either express or implied.
% See the License for the specific language governing permissions and
% limitations under the License.

function vel_k_h_W    = fcn(vel_k_O,ENVMT)
%fcn - Calculate horizontal kinetic velocity in wind reference frame
%
% Inputs:
%    vel_k_O    - Kinetic velocity in inertial reference frame
%    ENVMT      - Environment characteristics
%
% Outputs:
%    vel_k_h_W  - Horizontal kinetic velocity magnitude in wind reference frame
%
%
% Author: Sebastian Rapp, Ph.D., Revised by: Dylan Eijkelhof, M.Sc.
% Delft University of Technology
% email address: s.rapp@tudelft.nl
% email address: d.eijkelhof@tudelft.nl
% December 2019; Last revision: 06-October-2020

%-------------	BEGIN CODE	--------------

vel_k_W = transformFromOtoW(ENVMT.windDirection_rad, vel_k_O);

vel_k_h_W = sign(-vel_k_W(1))*sqrt( vel_k_W(1)^2 + vel_k_W(2)^2 );

%-------------	 END CODE	--------------
end

== matlab function Dyn_6DoF_v2_0_R2015B/AirborneSystem/FlightControlSystem/PathFollowingController_SS_3/FlightOnFlatEarth (Retraction&Loitering)/CalculateAttitudeCmds/FlightPathLoopRetraction_Aerodynamic/PIController_opt/wrapCourse ==
  data: chi_ref input; e_course output; chi input
% Copyright 2021 Delft University of Technology
%
% Licensed under the Apache License, Version 2.0 (the "License");
% you may not use this file except in compliance with the License.
% You may obtain a copy of the License at
%
%      http://www.apache.org/licenses/LICENSE-2.0
%
% Unless required by applicable law or agreed to in writing, software
% distributed under the License is distributed on an "AS IS" BASIS,
% WITHOUT WARRANTIES OR CONDITIONS OF ANY KIND, either express or implied.
% See the License for the specific language governing permissions and
% limitations under the License.

function e_course = course_error(chi_ref, chi)
%course_error - Calculate the error between commanded and actual course angle
%
% Inputs:
%    chi_ref  - Required chi
%    chi      - Actual chi
%
% Outputs:
%    e_course - Course (heading) error
%
% Author: Sebastian Rapp, Ph.D., Revised by: Dylan Eijkelhof, M.Sc.
% Delft University of Technology
% email address: s.rapp@tudelft.nl
% email address: d.eijkelhof@tudelft.nl
% December 2019; Last revision: 06-October-2020

%-------------	BEGIN CODE	--------------

%#codegen
% The vectors are lying in the tangential plane attached to the current
% position on the small earth.
p_bearing_vec =   [cos(chi);         sin(chi);         0];
p_bearing_vec = p_bearing_vec/norm(p_bearing_vec); 
ref_bearing_vec = [cos(chi_ref); sin(chi_ref); 0];
ref_bearing_vec = ref_bearing_vec/norm(ref_bearing_vec); 

e_z = cross( ref_bearing_vec, p_bearing_vec ); 

dot_product = dot( ref_bearing_vec, p_bearing_vec ); 
if dot_product > 1 
    dot_product = 1; 
end
if dot_product < -1 
    dot_product = -1; 
end

e_course = - sign( e_z(3) ) * acos( dot_product );
%-------------	 END CODE	--------------
end
